simulink subsystem "Simulator_MID_v4"  (R2023a)
settings: Solver=VariableStepAuto  StartTime=0.0  StopTime=10.0  RelTol=1e-3
model mask{rho=971, c_p=4179, pi=3.14151, f_Darcy=0.025, L_F=40, D_F=0.4, h_F=1.5, D_S1=0.1, L_S1=5, h_S1=1.5, D_S2=0.02, L_S2=50, h_S2=1.5, D_S3=0.1, L_S3=5, h_S3=1.5, D_R=0.4, L_R=40, h_R=1.5, C_b=300000000, A_b=500, h_b=1.5, L_BYP=0, D_BYP=0, h_BYP=1.5, T_F_0=350, T_S1_0=283, T_S2_0=283, T_S3_0=283, T_b_0=300, T_R_0=283, T_BYP_0=283}
  mask prompts: rho "rho water [kg/m^3]"; c_p "c_p water [J/kgK]"; f_Darcy "Darcy friction factor"; L_F "Length of F [m]"; D_F "Diameter of F [m]"; h_F "h_F [W/m^2K]"; D_S1 "Diameter of S1 [m]"; L_S1 "Length of S1  [m]"; h_S1 "h_S1 [W/m^2K]"; D_S2 "Diameter of S2  [m]"; L_S2 "Length of S2  [m]"; h_S2 "h_S2 [W/m^2K]"; D_S3 "Diameter of S3  [m]"; L_S3 "Length of S3  [m]"; h_S3 "h_S3 [W/m^2K]"; D_R "Diameter of R  [m]"; L_R "Length of R  [m]"; h_R "h_R [W/m^2K]"; C_b "C_building [J/K]"; A_b "A_building_hull  [m^2]"; h_b "h_building [W/m^2K]"; L_BYP "[NOT USED]"; D_BYP "[NOT USED]"; h_BYP "[NOT USED]"; T_F_0 "T_F_0 [K]"; T_S1_0 "T_S1_0 [K]"; T_S2_0 "T_S2_0 [K]"; T_S3_0 "T_S3_0 [K]"; T_b_0 "T_b_0 [K]"; T_R_0 "T_R_0 [K]"; T_BYP_0 "[NOT USED]"
undefined symbols (not defined in the file): C_F, C_R, C_S1, C_S2, C_S3, k_b, k_F, k_R, k_S1, k_S2, k_S3
settings Model: Creator=alex  LastModifiedBy=alex
settings OptimizationCC: ReuseModelBlockBuffer=off

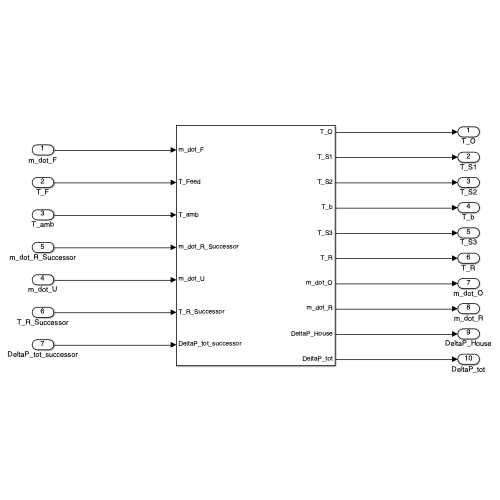
[thumbnail: Simulink's stored preview of the top-level diagram]
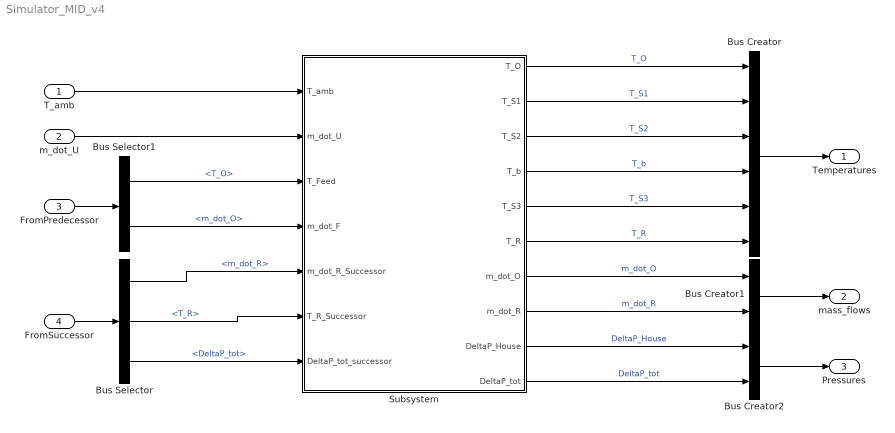
== system Simulator_MID_v4 ==
  T_amb : Inport
  m_dot_U : Inport  Port=2
  FromPredecessor : Inport  Port=3
  FromSuccessor : Inport  Port=4
  Bus Creator : BusCreator  Inputs=6
  Bus Creator1 : BusCreator  Inputs=2
  Bus Creator2 : BusCreator  Inputs=2
  Bus Selector : BusSelector  OutputSignals=m_dot_R,T_R,DeltaP_tot
  Bus Selector1 : BusSelector  OutputSignals=T_O,m_dot_O
  Subsystem : Subsystem
  Temperatures : Outport
  mass_flows : Outport  Port=2
  Pressures : Outport  Port=3
  wires:
  T_amb/1 -> Subsystem/1(T_amb)
  m_dot_U/1 -> Subsystem/2(m_dot_U)
  Subsystem/9(DeltaP_House) -> Bus Creator2/1  "DeltaP_House"
  Subsystem/3(T_S2) -> Bus Creator/3  "T_S2"
  Subsystem/6(T_R) -> Bus Creator/6  "T_R"
  Subsystem/5(T_S3) -> Bus Creator/5  "T_S3"
  Subsystem/4(T_b) -> Bus Creator/4  "T_b"
  Subsystem/10(DeltaP_tot) -> Bus Creator2/2  "DeltaP_tot"
  Subsystem/7(m_dot_O) -> Bus Creator1/1  "m_dot_O"
  Subsystem/1(T_O) -> Bus Creator/1  "T_O"
  Subsystem/8(m_dot_R) -> Bus Creator1/2  "m_dot_R"
  Subsystem/2(T_S1) -> Bus Creator/2  "T_S1"
  Bus Creator/1 -> Temperatures/1
  Bus Creator1/1 -> mass_flows/1
  Bus Creator2/1 -> Pressures/1
  Bus Selector/1 -> Subsystem/5(m_dot_R_Successor)  "<m_dot_R>"
  Bus Selector/2 -> Subsystem/6(T_R_Successor)  "<T_R>"
  FromSuccessor/1 -> Bus Selector/1
  FromPredecessor/1 -> Bus Selector1/1
  Bus Selector/3 -> Subsystem/7(DeltaP_tot_successor)  "<DeltaP_tot>"
  Bus Selector1/1 -> Subsystem/3(T_Feed)  "<T_O>"
  Bus Selector1/2 -> Subsystem/4(m_dot_F)  "<m_dot_O>"

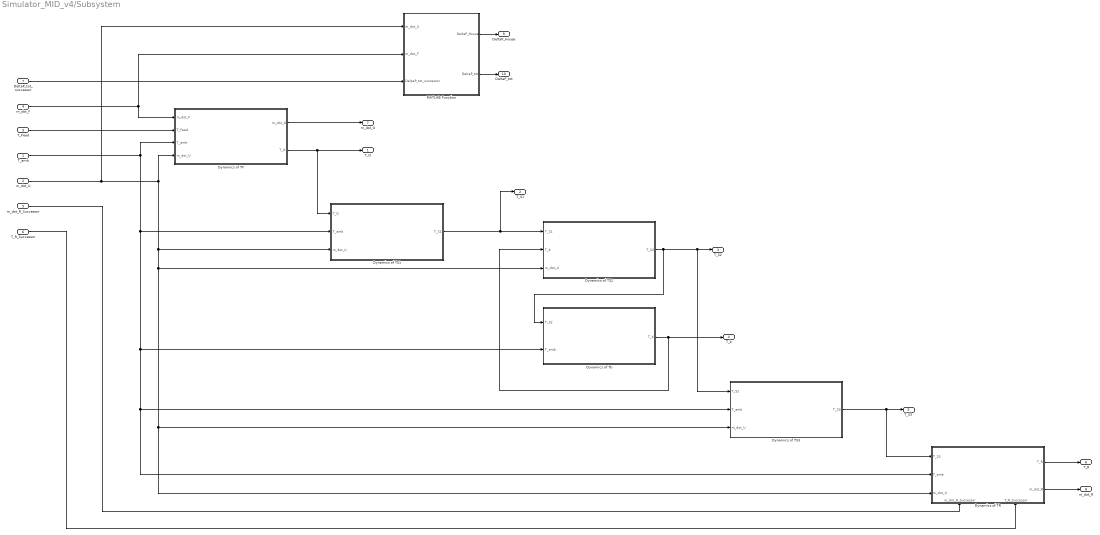
== system Simulator_MID_v4/Subsystem ==
  T_amb : Inport
  m_dot_U : Inport  Port=2
  T_Feed : Inport  Port=3
  m_dot_F : Inport  Port=4
  m_dot_R_Successor : Inport  Port=5
  T_R_Successor : Inport  Port=6
  DeltaP_tot_successor : Inport  Port=7
  Dynamics of TF : Subsystem
  Dynamics of TR : Subsystem
      settings: PortSchema="{\"entries\":[{\"content\":{\"sides\":[{\"content\":{\"connectorIds\":[\"In1\",\"In2\",\"In3\"]},\"type\":\"ConnectorPlacement.EquallySpacedRectSide\",\"uuid\":\"1d5cfb0c-3444-494a-8f15-ea1ce9aa89e1\"},{\"content\":{\"connectorIds\":[\"Out1\",\"Out2\"],\"side\":\"RIGHT\"},\"type\":\"ConnectorPlacement.EquallySpacedRectSide\",\"uuid\":\"a241c28b-af63-4b6d-8a8e-9e454c2f304f\"},{\"content\":{\"side\":\"TOP\"},\"type\":\"ConnectorPlacement.EquallySpacedRectSide\",\"uuid\":\"7a4239f2-e3be-4ccc-ba79-85038cac89dd\"},{\"content\":{\"connectorIds\":[\"In4\",\"In5\"],\"side\":\"BOTTOM\"},\"type\":\"ConnectorPlacement.EquallySpacedRectSide\",\"uuid\":\"03da5dbc-12e1-4117-b594-812fe8cbcf6d\"}]},\"type\":\"ConnectorPlacement.EquallySpacedConnector\",\"uuid\":\"6bf2d3a5-b163-467e-ac11-ed480dce725b\"}],\"packageUris\":[\"http://schema.mathworks.com/mf0/Connector/R2020b\"],\"version\":\"1.0\"}"
  Dynamics of TS1 : Subsystem
  Dynamics of TS2 : Subsystem
  Dynamics of TS3 : Subsystem
  Dynamics of Tb : Subsystem
  MATLAB Function : MATLAB Function  TreatAsAtomicUnit=on
  T_O : Outport
  T_S1 : Outport  Port=2
  T_S2 : Outport  Port=3
  T_b : Outport  Port=4
  T_S3 : Outport  Port=5
  T_R : Outport  Port=6
  m_dot_O : Outport  Port=7
  m_dot_R : Outport  Port=8
  DeltaP_House : Outport  Port=9
  DeltaP_tot : Outport  Port=10
  wires:
  MATLAB Function/2(DeltaP_tot) -> DeltaP_tot/1
  m_dot_F/1 -> MATLAB Function/2(m_dot_F), Dynamics of TF/1(m_dot_F)
  T_Feed/1 -> Dynamics of TF/2(T_Feed)
  T_amb/1 -> Dynamics of Tb/2(T_amb), Dynamics of TS3/2(T_amb), Dynamics of TR/2(T_amb), Dynamics of TS1/2(T_amb), Dynamics of TF/3(T_amb)
  m_dot_U/1 -> Dynamics of TR/3(m_dot_U), Dynamics of TS3/3(m_dot_U), Dynamics of TS2/3(m_dot_U), Dynamics of TS1/3(m_dot_U), Dynamics of TF/4(m_dot_U), MATLAB Function/1(m_dot_U)
  Dynamics of TF/1(m_dot_O) -> m_dot_O/1
  Dynamics of TF/2(T_O) -> Dynamics of TS1/1(T_O), T_O/1
  Dynamics of TS1/1(T_S1) -> T_S1/1, Dynamics of TS2/1(T_S1)
  Dynamics of TS2/1(T_S2) -> T_S2/1, Dynamics of TS3/1(T_S2), Dynamics of Tb/1(T_S2)
  Dynamics of Tb/1(T_b) -> T_b/1, Dynamics of TS2/2(T_b)
  m_dot_R_Successor/1 -> Dynamics of TR/4(m_dot_R_Successor)
  T_R_Successor/1 -> Dynamics of TR/5(T_R_Successor)
  Dynamics of TS3/1(T_S3) -> T_S3/1, Dynamics of TR/1(T_S3)
  Dynamics of TR/1(T_R) -> T_R/1
  Dynamics of TR/2(m_dot_R) -> m_dot_R/1
  MATLAB Function/1(DeltaP_House) -> DeltaP_House/1
  DeltaP_tot_successor/1 -> MATLAB Function/3(DelpaP_tot_successor)

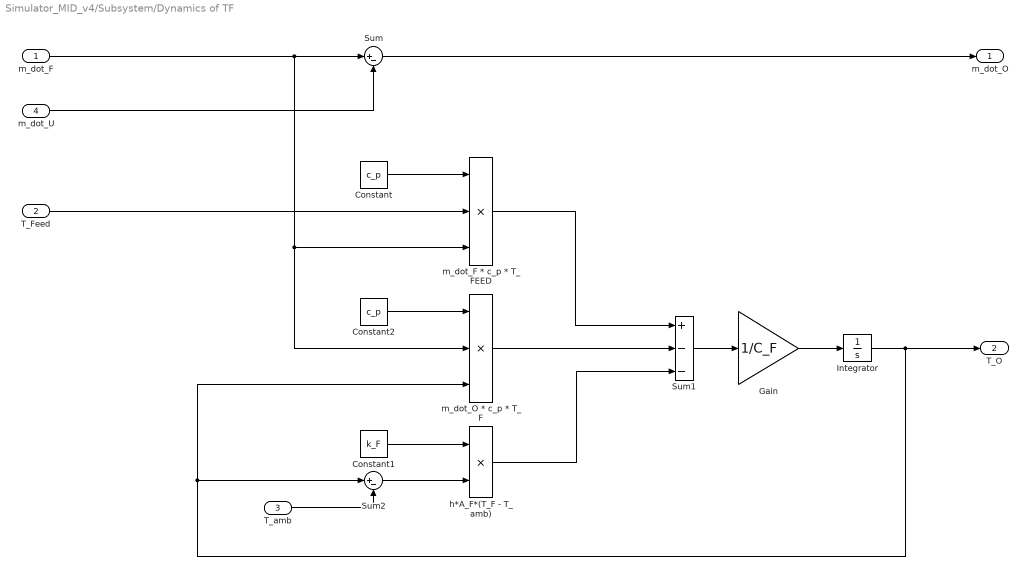
== system Simulator_MID_v4/Subsystem/Dynamics of TF ==
  m_dot_F : Inport
  T_Feed : Inport  Port=2
  T_amb : Inport  Port=3
  m_dot_U : Inport  Port=4
  Constant : Constant  Value=c_p
  Constant1 : Constant  Value=k_F
  Constant2 : Constant  Value=c_p
  Gain : Gain  Gain=1/C_F
  Integrator : Integrator  InitialCondition=T_F_0
  Sum : Sum  Inputs=|+-
  Sum1 : Sum  Inputs=+--
  Sum2 : Sum  Inputs=|+-
  h*A_F*(T_F - T_amb) : Product
  m_dot_F * c_p * T_FEED : Product  Inputs=3
  m_dot_O * c_p * T_F : Product  Inputs=3
  m_dot_O : Outport
  T_O : Outport  Port=2
  wires:
  Constant2/1 -> m_dot_O * c_p * T_F/1
  m_dot_O * c_p * T_F/1 -> Sum1/2
  T_amb/1 -> Sum2/2
  Integrator/1 -> T_O/1, m_dot_O * c_p * T_F/3, Sum2/1
  Constant1/1 -> h*A_F*(T_F - T_amb)/1
  h*A_F*(T_F - T_amb)/1 -> Sum1/3
  Sum2/1 -> h*A_F*(T_F - T_amb)/2
  m_dot_F * c_p * T_FEED/1 -> Sum1/1
  Constant/1 -> m_dot_F * c_p * T_FEED/1
  Sum1/1 -> Gain/1
  m_dot_F/1 -> m_dot_F * c_p * T_FEED/3, m_dot_O * c_p * T_F/2, Sum/1
  Gain/1 -> Integrator/1
  Sum/1 -> m_dot_O/1
  T_Feed/1 -> m_dot_F * c_p * T_FEED/2
  m_dot_U/1 -> Sum/2

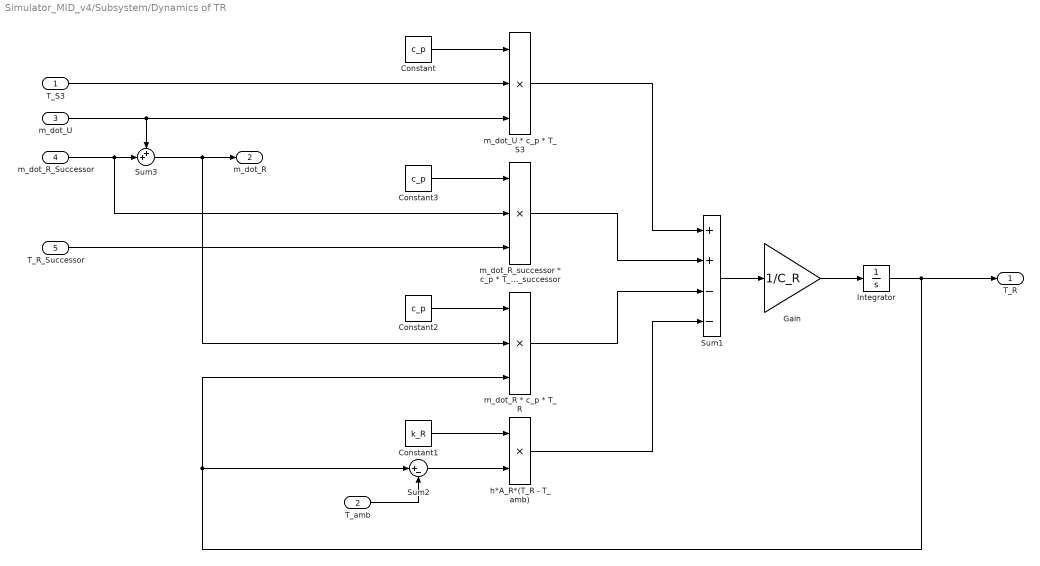
== system Simulator_MID_v4/Subsystem/Dynamics of TR ==
  T_S3 : Inport
  T_amb : Inport  Port=2
  m_dot_U : Inport  Port=3
  m_dot_R_Successor : Inport  Port=4
  T_R_Successor : Inport  Port=5
  Constant : Constant  Value=c_p
  Constant1 : Constant  Value=k_R
  Constant2 : Constant  Value=c_p
  Constant3 : Constant  Value=c_p
  Gain : Gain  Gain=1/C_R
  Integrator : Integrator  InitialCondition=T_R_0
  Sum1 : Sum  Inputs=++--
  Sum2 : Sum  Inputs=|+-
  Sum3 : Sum  Inputs=++|
  h*A_R*(T_R - T_amb) : Product
  m_dot_R * c_p * T_R : Product  Inputs=3
  m_dot_R_successor * c_p * T_R_successor : Product  Inputs=3
  m_dot_U * c_p * T_S3 : Product  Inputs=3
  T_R : Outport
  m_dot_R : Outport  Port=2
  wires:
  Constant2/1 -> m_dot_R * c_p * T_R/1
  T_amb/1 -> Sum2/2
  Integrator/1 -> T_R/1, m_dot_R * c_p * T_R/3, Sum2/1
  Constant1/1 -> h*A_R*(T_R - T_amb)/1
  Sum2/1 -> h*A_R*(T_R - T_amb)/2
  Constant/1 -> m_dot_U * c_p * T_S3/1
  Sum1/1 -> Gain/1
  Gain/1 -> Integrator/1
  T_S3/1 -> m_dot_U * c_p * T_S3/2
  m_dot_U/1 -> m_dot_U * c_p * T_S3/3, Sum3/1
  Sum3/1 -> m_dot_R * c_p * T_R/2, m_dot_R/1
  m_dot_R_Successor/1 -> m_dot_R_successor * c_p * T_R_successor/2, Sum3/2
  Constant3/1 -> m_dot_R_successor * c_p * T_R_successor/1
  T_R_Successor/1 -> m_dot_R_successor * c_p * T_R_successor/3
  h*A_R*(T_R - T_amb)/1 -> Sum1/4
  m_dot_R * c_p * T_R/1 -> Sum1/3
  m_dot_R_successor * c_p * T_R_successor/1 -> Sum1/2
  m_dot_U * c_p * T_S3/1 -> Sum1/1

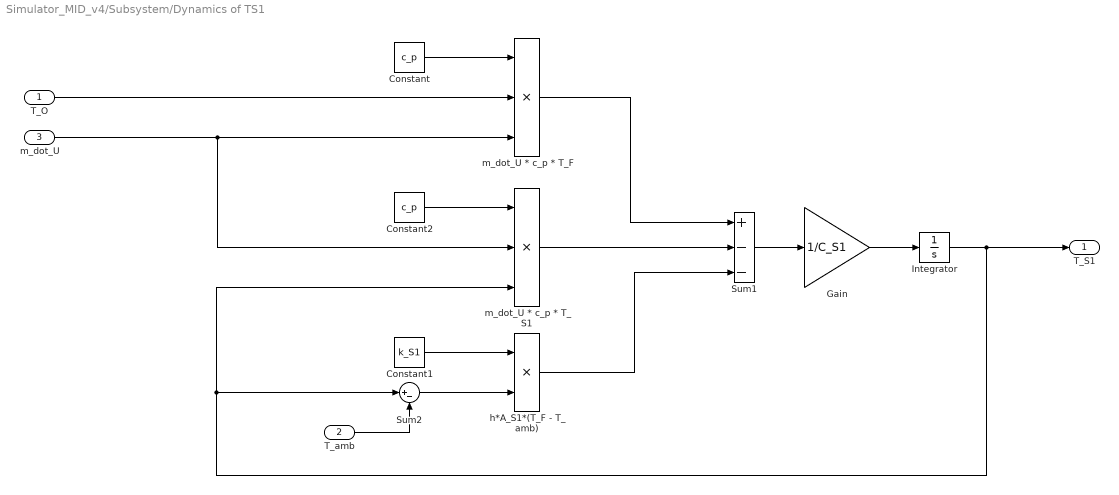
== system Simulator_MID_v4/Subsystem/Dynamics of TS1 ==
  T_O : Inport
  T_amb : Inport  Port=2
  m_dot_U : Inport  Port=3
  Constant : Constant  Value=c_p
  Constant1 : Constant  Value=k_S1
  Constant2 : Constant  Value=c_p
  Gain : Gain  Gain=1/C_S1
  Integrator : Integrator  InitialCondition=T_S1_0
  Sum1 : Sum  Inputs=+--
  Sum2 : Sum  Inputs=|+-
  h*A_S1*(T_F - T_amb) : Product
  m_dot_U * c_p * T_F : Product  Inputs=3
  m_dot_U * c_p * T_S1 : Product  Inputs=3
  T_S1 : Outport
  wires:
  Constant2/1 -> m_dot_U * c_p * T_S1/1
  m_dot_U * c_p * T_S1/1 -> Sum1/2
  T_amb/1 -> Sum2/2
  Integrator/1 -> T_S1/1, m_dot_U * c_p * T_S1/3, Sum2/1
  Constant1/1 -> h*A_S1*(T_F - T_amb)/1
  h*A_S1*(T_F - T_amb)/1 -> Sum1/3
  Sum2/1 -> h*A_S1*(T_F - T_amb)/2
  m_dot_U * c_p * T_F/1 -> Sum1/1
  Constant/1 -> m_dot_U * c_p * T_F/1
  Sum1/1 -> Gain/1
  Gain/1 -> Integrator/1
  T_O/1 -> m_dot_U * c_p * T_F/2
  m_dot_U/1 -> m_dot_U * c_p * T_S1/2, m_dot_U * c_p * T_F/3

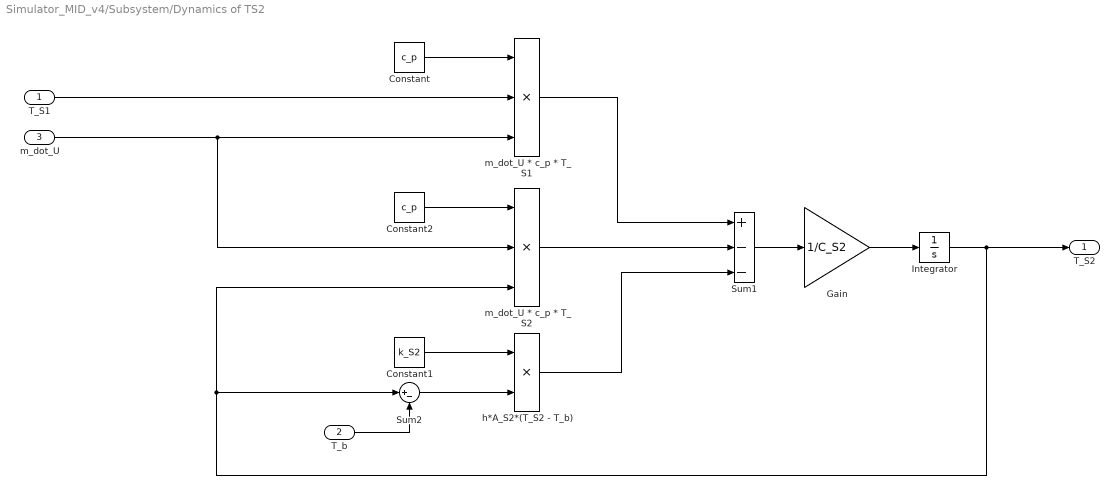
== system Simulator_MID_v4/Subsystem/Dynamics of TS2 ==
  T_S1 : Inport
  T_b : Inport  Port=2
  m_dot_U : Inport  Port=3
  Constant : Constant  Value=c_p
  Constant1 : Constant  Value=k_S2
  Constant2 : Constant  Value=c_p
  Gain : Gain  Gain=1/C_S2
  Integrator : Integrator  InitialCondition=T_S2_0
  Sum1 : Sum  Inputs=+--
  Sum2 : Sum  Inputs=|+-
  h*A_S2*(T_S2 - T_b) : Product
  m_dot_U * c_p * T_S1 : Product  Inputs=3
  m_dot_U * c_p * T_S2 : Product  Inputs=3
  T_S2 : Outport
  wires:
  Constant2/1 -> m_dot_U * c_p * T_S2/1
  m_dot_U * c_p * T_S2/1 -> Sum1/2
  T_b/1 -> Sum2/2
  Constant1/1 -> h*A_S2*(T_S2 - T_b)/1
  h*A_S2*(T_S2 - T_b)/1 -> Sum1/3
  Sum2/1 -> h*A_S2*(T_S2 - T_b)/2
  m_dot_U * c_p * T_S1/1 -> Sum1/1
  Constant/1 -> m_dot_U * c_p * T_S1/1
  Sum1/1 -> Gain/1
  Gain/1 -> Integrator/1
  m_dot_U/1 -> m_dot_U * c_p * T_S2/2, m_dot_U * c_p * T_S1/3
  Integrator/1 -> T_S2/1, Sum2/1, m_dot_U * c_p * T_S2/3
  T_S1/1 -> m_dot_U * c_p * T_S1/2

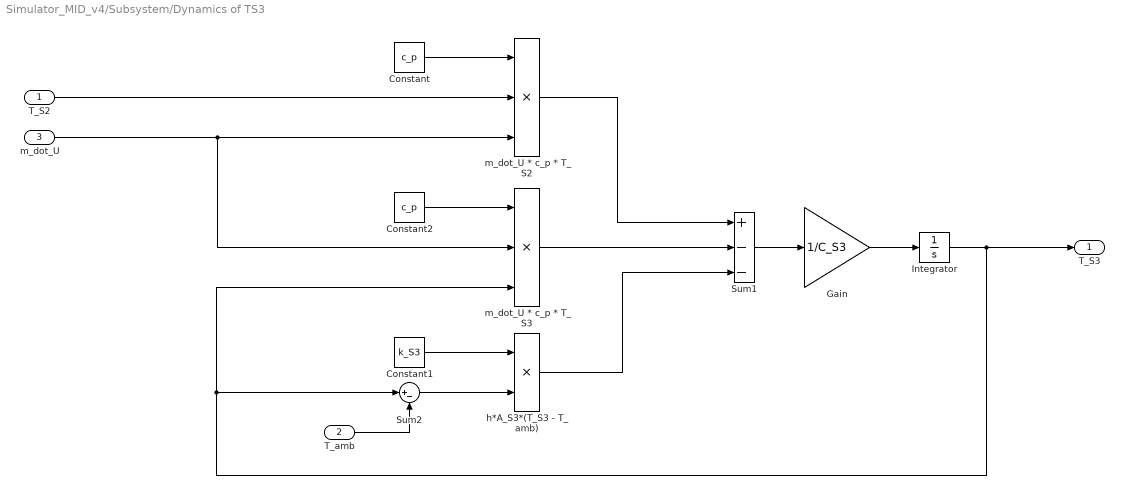
== system Simulator_MID_v4/Subsystem/Dynamics of TS3 ==
  T_S2 : Inport
  T_amb : Inport  Port=2
  m_dot_U : Inport  Port=3
  Constant : Constant  Value=c_p
  Constant1 : Constant  Value=k_S3
  Constant2 : Constant  Value=c_p
  Gain : Gain  Gain=1/C_S3
  Integrator : Integrator  InitialCondition=T_S3_0
  Sum1 : Sum  Inputs=+--
  Sum2 : Sum  Inputs=|+-
  h*A_S3*(T_S3 - T_amb) : Product
  m_dot_U * c_p * T_S2 : Product  Inputs=3
  m_dot_U * c_p * T_S3 : Product  Inputs=3
  T_S3 : Outport
  wires:
  Constant2/1 -> m_dot_U * c_p * T_S3/1
  m_dot_U * c_p * T_S3/1 -> Sum1/2
  T_amb/1 -> Sum2/2
  Integrator/1 -> T_S3/1, m_dot_U * c_p * T_S3/3, Sum2/1
  Constant1/1 -> h*A_S3*(T_S3 - T_amb)/1
  h*A_S3*(T_S3 - T_amb)/1 -> Sum1/3
  Sum2/1 -> h*A_S3*(T_S3 - T_amb)/2
  m_dot_U * c_p * T_S2/1 -> Sum1/1
  Constant/1 -> m_dot_U * c_p * T_S2/1
  Sum1/1 -> Gain/1
  Gain/1 -> Integrator/1
  T_S2/1 -> m_dot_U * c_p * T_S2/2
  m_dot_U/1 -> m_dot_U * c_p * T_S3/2, m_dot_U * c_p * T_S2/3

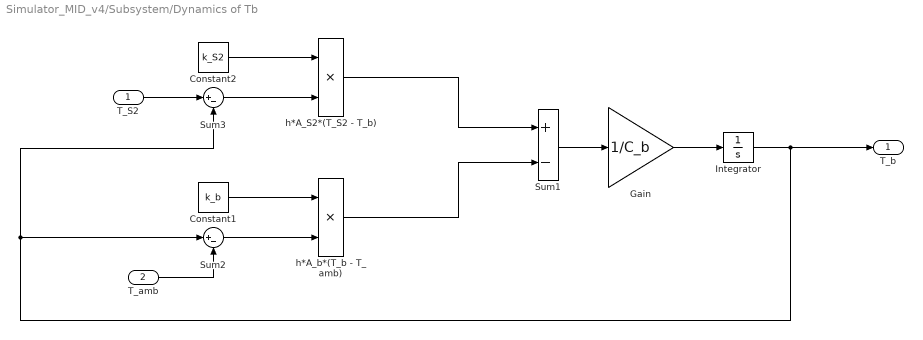
== system Simulator_MID_v4/Subsystem/Dynamics of Tb ==
  T_S2 : Inport
  T_amb : Inport  Port=2
  Constant1 : Constant  Value=k_b
  Constant2 : Constant  Value=k_S2
  Gain : Gain  Gain=1/C_b
  Integrator : Integrator  InitialCondition=T_b_0
  Sum1 : Sum  Inputs=+-
  Sum2 : Sum  Inputs=|+-
  Sum3 : Sum  Inputs=|+-
  h*A_S2*(T_S2 - T_b) : Product
  h*A_b*(T_b - T_amb) : Product
  T_b : Outport
  wires:
  T_amb/1 -> Sum2/2
  Integrator/1 -> T_b/1, Sum3/2, Sum2/1
  Constant1/1 -> h*A_b*(T_b - T_amb)/1
  Sum2/1 -> h*A_b*(T_b - T_amb)/2
  Sum1/1 -> Gain/1
  Gain/1 -> Integrator/1
  Sum3/1 -> h*A_S2*(T_S2 - T_b)/2
  Constant2/1 -> h*A_S2*(T_S2 - T_b)/1
  h*A_b*(T_b - T_amb)/1 -> Sum1/2
  T_S2/1 -> Sum3/1
  h*A_S2*(T_S2 - T_b)/1 -> Sum1/1

== matlab function Simulator_MID_v4/Subsystem/MATLAB Function ==
  data: DeltaP_House output; m_dot_U input; m_dot_F input; f_Darcy parameter; L_S1 parameter; L_S2 parameter; L_S3 parameter; L_F parameter; L_R parameter; D_S1 parameter; D_S2 parameter; D_S3 parameter; D_F parameter; D_R parameter; rho parameter; pi parameter; DeltaP_tot output; DelpaP_tot_successor input
function [DeltaP_House,DeltaP_tot] = fcn(m_dot_U, m_dot_F, f_Darcy, L_S1, L_S2, L_S3, L_F, L_R, D_S1, D_S2, D_S3, D_F, D_R, rho, pi, DelpaP_tot_successor)
      DeltaP_S1= 8*f_Darcy*L_S1*m_dot_U^2/(rho*pi^2*D_S1^5);
      DeltaP_S2= 8*f_Darcy*L_S2*m_dot_U^2/(rho*pi^2*D_S2^5); 
      DeltaP_S3= 8*f_Darcy*L_S3*m_dot_U^2/(rho*pi^2*D_S3^5); 
      DeltaP_F= 8*f_Darcy*L_F*m_dot_F^2/(rho*pi^2*D_F^5); 
      DeltaP_R= 8*f_Darcy*L_R*m_dot_F^2/(rho*pi^2*D_R^5); 
      
      DeltaP_S1_S2_S3 = DeltaP_S1+DeltaP_S2+DeltaP_S3;
      DeltaP_House = max(DeltaP_S1_S2_S3, DelpaP_tot_successor);

      DeltaP_tot = DeltaP_House+DeltaP_F+DeltaP_R;
